simulink model "LineDetectionDSK6416"  (Simulink 6.5)
settings: Solver=FixedStepDiscrete  SolverMode=SingleTasking  StartTime=0.0  StopTime=inf  RelTol=1e-3
libraries: rtdxBlocks x2, viptransforms x2, dspindex x2, c6000tgtpreflib x1, vipconversions x1, vipanalysis x1, vipstatistics x1, viptextngfix x1
settings Model: Creator=jfaing  LastModifiedBy=JacobF  ProdHWDeviceType=TI C6000
settings SolverCC: PositivePriorityOrder=on
settings DataIOCC: SaveOutput=off  SaveTime=off
settings OptimizationCC: OptimizeModelRefInitCode=on
settings HardwareCC: ProdBitPerLong=40  ProdIntDivRoundTo=Zero  ProdEndianess=LittleEndian  ProdHWDeviceType=TI C6000  TargetHWDeviceType=32-bit Generic
settings RTWCC: SystemTargetFile=ti_c6000_ert.tlc  GenCodeOnly=on  TemplateMakefile=ti_c6000_ert.tmf  Description=Embedded Target for TI C6000 DSP (ERT)  ProcessScript=ti_c6000_ert_make_rtw_hook
settings CodeAppCC: IgnoreCustomStorageClasses=off
settings C6000ERTTargetCC: TargetFcnLib=ansi_tfl_tmw.mat  GenFloatMathFcnCalls=ANSI_C  UtilityFuncGeneration=Auto  GenerateFullHeader=on  GenerateSampleERTMain=off  GenerateTestInterfaces=off  IsPILTarget=off  ModelReferenceCompliant=on  IncludeMdlTerminateFcn=on  CombineOutputUpdateFcns=on  SuppressErrorStatus=off  IncludeFileDelimiter=Auto  ERTCustomFileBanners=on  SupportAbsoluteTime=on  LogVarNameModifier=rt_  MatFileLogging=off  MultiInstanceERTCode=off  SupportNonFinite=on  SupportComplex=on  PurelyIntegerCode=off  SupportContinuousTime=off  SupportNonInlinedSFcns=off  EnableShiftOperators=on  ParenthesesLevel=Nominal  GenerateErtSFunction=off  GenerateASAP2=off  ExtMode=off  ExtModeTransport=0  ExtModeStaticAlloc=off  ExtModeStaticAllocSize=1000000  ExtModeTesting=off  ExtModeMexFile=ext_comm  InlinedParameterPlacement=NonHierarchical  TargetOS=BareBoardExample  MultiInstanceErrorCode=Error  RateGroupingCode=on  RootIOFormat=Individual arguments  RTWCAPISignals=off  RTWCAPIParams=off  RTWCAPIStates=off  ERTSrcFileBannerTemplate=ert_code_template.cgt  ERTHdrFileBannerTemplate=ert_code_template.cgt  ERTDataSrcFileTemplate=ert_code_template.cgt  ERTDataHdrFileTemplate=ert_code_template.cgt  ERTCustomFileTemplate=example_file_process.tlc  ModuleNamingRule=Unspecified  SignalDisplayLevel=10  ParamTuneLevel=10  GlobalDataDefinition=Auto  DataDefinitionFile=global.c  GlobalDataReference=Auto  DataReferenceFile=global.h  GRTInterface=off  EnableUserReplacementTypes=off  MemSecPackage=--- None ---  MemSecDataConstants=Default  MemSecDataIO=Default  MemSecDataInternal=Default  MemSecDataParameters=Default  MemSecFuncInitTerm=Default  MemSecFuncExecute=Default  exportCCSObj=on  ccsObjName=CCS_Obj  useDSPBIOS=off  ProfileGenCode=off  InlineDSPBlks=on  FPopt=off  memModel=Far_Aggregate  optLevel=Function(-o2)  CompilerVerbosity=Quiet  InterruptThreshOnC6x=off  SymbolicDebugOnC6x=off  RetainAsmFiles=off  RetainObjFiles=off  CreateMapFile=off  UserStackSize=8192  c6000BuildAction=Create_CCS_Project  OverrunAction=Notify_and_continue  OverrunNotificationMethod=Turn_on_LEDs

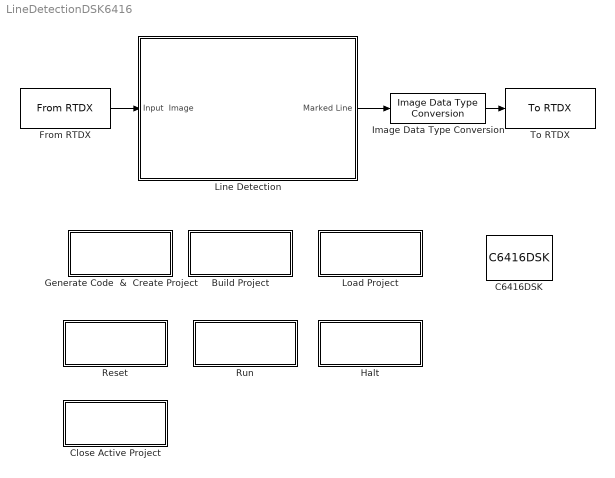
== system LineDetectionDSK6416 ==
  Build Project : Subsystem
      settings: OpenFcn=CCS_Obj.build;
      mask Display: disp('Build\nProject')
  C6416DSK : c6000tgtpreflib/C6416DSK  Tag=C6000 TARGET PREFERENCES BLOCK  SystemSampleTime=-1
  Close Active Project : Subsystem
      settings: OpenFcn=close(CCS_Obj,[],'project')
      mask Display: disp('Close Active Project')
  From RTDX : rtdxBlocks/From RTDX  channelNameStr=inputimage  isBlocking=on  icMaskVar=0  Ts=-1  dims=[99 101]  isFrame=off  dType=uint8  isChannelEnabled=on  isHighSpeedRTDXUsed=on
  Generate Code  &  Create Project : Subsystem
      settings: OpenFcn=make_rtw;
      mask Display: disp('Generate Code\n & \nCreate Project')
  Halt : Subsystem
      settings: OpenFcn=CCS_Obj.halt;
      mask Display: disp('Halt')
  Image Data Type Conversion : vipconversions/Image Data Type Conversion  outDT=uint8  isSigned=on  wordLen=16  numFracBits=0
  Line Detection : Subsystem
  Load Project : Subsystem
      settings: OpenFcn=CCS_Obj.load([pwd,'\',bdroot,'_c6000_rtw\', bdroot, '.out'])
      mask Display: disp('Load\nProject')
  Reset : Subsystem
      settings: OpenFcn=CCS_Obj.reset;
      mask Display: disp('Reset')
  Run : Subsystem
      settings: OpenFcn=CCS_Obj.run;
      mask Display: disp('Run')
  To RTDX : rtdxBlocks/To RTDX  channelNameStr=outputimage  isBlocking=on  isChannelEnabled=on
  wires:
  Image Data Type Conversion/1 -> To RTDX/1
  From RTDX/1 -> Line Detection/1(Input  Image)
  Line Detection/1(Marked Line) -> Image Data Type Conversion/1

== system LineDetectionDSK6416/Build Project ==

== system LineDetectionDSK6416/Close Active Project ==

== system LineDetectionDSK6416/Generate Code  &  Create Project ==

== system LineDetectionDSK6416/Halt ==

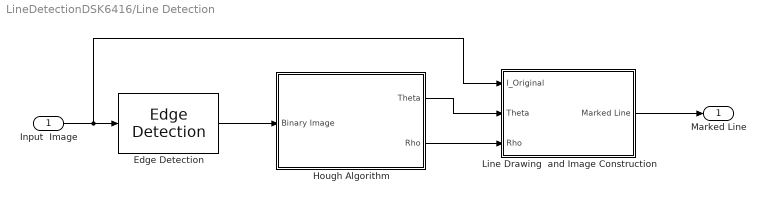
== system LineDetectionDSK6416/Line Detection ==
  Input  Image : Inport
  Edge Detection : vipanalysis/Edge Detection  DialogController=vipDDGCreate  DialogControllerArgs=DataTag1  method=Sobel  outputType=Binary image  userDefinedThreshold=on  thresholdSource=Specify via dialog  threshold=20  thresholdTuning=4  edgeThinning=off  threshold_canny=[0.25 0.60]  autoPercent=70  sigma=1  prodOutputMode=Binary point scaling  prodOutputWordLength=32  prodOutputFracLength=8  roundingMode=Floor  overflowMode=off
  Hough Algorithm : Subsystem
  Line Drawing  and Image Construction : Subsystem
  Marked Line : Outport
  wires:
  Edge Detection/1 -> Hough Algorithm/1(Binary Image)
  Hough Algorithm/2(Rho) -> Line Drawing  and Image Construction/3(Rho)
  Line Drawing  and Image Construction/1(Marked Line) -> Marked Line/1
  Hough Algorithm/1(Theta) -> Line Drawing  and Image Construction/2(Theta)
  Input  Image/1 -> Edge Detection/1, Line Drawing  and Image Construction/1(I_Original)

== system LineDetectionDSK6416/Load Project ==

== system LineDetectionDSK6416/Reset ==

== system LineDetectionDSK6416/Run ==

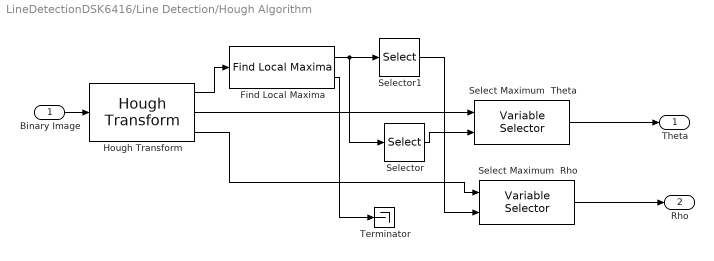
== system LineDetectionDSK6416/Line Detection/Hough Algorithm ==
  Binary Image : Inport
  Find Local Maxima : vipstatistics/Find Local Maxima  num_peaks=1  nhood_size=[5 7]  src_thresh=Specify via dialog  threshold=10  inputIsHough=on  dt_peak=uint32  dt_count=uint32
  Hough Transform : viptransforms/Hough Transform  DialogController=vipDDGCreate  DialogControllerArgs=DataTag2  theta_res=pi/360  rho_res=1  out_theta_rho=on  outdtmode=double  firstCoeffMode=Binary point scaling  firstCoeffWordLength=16  firstCoeffFracLength=14  secondCoeffMode=Binary point scaling  secondCoeffWordLength=32  secondCoeffFracLength=16  outputMode=Binary point scaling  outputWordLength=16  outputFracLength=0  accumMode=Binary point scaling  accumWordLength=32  accumFracLength=20  prodOutputMode=Binary point scaling  prodOutputWordLength=32  prodOutputFracLength=20  memoryMode=Binary point scaling  memoryWordLength=32  memoryFracLength=16  roundingMode=Nearest  overflowMode=on
  Select Maximum  Rho : dspindex/Variable Selector  NumInputs=1  rowsOrCols=Columns  IdxMode=Variable  Elements=[1 3]  ZerOneIdxMode=Zero-based  errmode=Clip Index  FillMode=on  FillValues=0
  Select Maximum  Theta : dspindex/Variable Selector  NumInputs=1  rowsOrCols=Columns  IdxMode=Variable  Elements=[1 3]  ZerOneIdxMode=Zero-based  errmode=Clip Index  FillMode=on  FillValues=0
  Selector : Selector  InputType=Vector  IndexMode=Zero-based  ElementSrc=Internal  Elements=1  RowSrc=Internal  Rows=1  ColumnSrc=Internal  Columns=1  InputPortWidth=2  IndexIsStartValue=off
  Selector1 : Selector  InputType=Vector  IndexMode=Zero-based  ElementSrc=Internal  Elements=0  RowSrc=Internal  Rows=1  ColumnSrc=Internal  Columns=1  InputPortWidth=2  IndexIsStartValue=off
  Terminator : Terminator
  Theta : Outport
  Rho : Outport  Port=2
  wires:
  Find Local Maxima/1 -> Selector1/1, Selector/1
  Find Local Maxima/2 -> Terminator/1
  Selector1/1 -> Select Maximum  Rho/2
  Selector/1 -> Select Maximum  Theta/2
  Hough Transform/3 -> Select Maximum  Rho/1
  Hough Transform/1 -> Find Local Maxima/1
  Hough Transform/2 -> Select Maximum  Theta/1
  Binary Image/1 -> Hough Transform/1
  Select Maximum  Theta/1 -> Theta/1
  Select Maximum  Rho/1 -> Rho/1

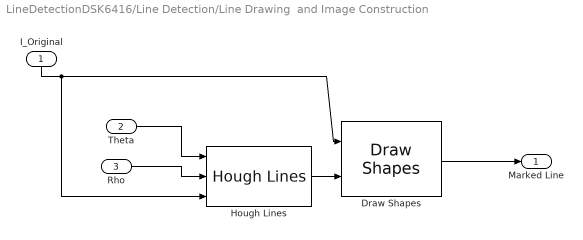
== system LineDetectionDSK6416/Line Detection/Line Drawing  and Image Construction ==
  I_Original : Inport  Orientation=down
  Theta : Inport  Port=2
  Rho : Inport  Port=3
  Draw Shapes : viptextngfix/Draw Shapes  DialogController=vipDDGCreate  DialogControllerArgs=DataTag3  inType=Intensity  shape=Lines  fill=off  display=White  intensity=200  color=[200 255 100]  opacity=0.6  viewport=Entire image  antialiasing=off
  Hough Lines : viptransforms/Hough Lines  DialogController=vipDDGCreate  DialogControllerArgs=DataTag4  sineCompMethod=Trigonometric function  thetaRes=pi/180  firstCoeffMode=Specify word length  firstCoeffWordLength=16  firstCoeffFracLength=15  prodOutputMode=Binary point scaling  prodOutputWordLength=32  prodOutputFracLength=16  roundingMode=Nearest  overflowMode=on
  Marked Line : Outport
  wires:
  Hough Lines/1 -> Draw Shapes/2
  I_Original/1 -> Draw Shapes/1, Hough Lines/3
  Theta/1 -> Hough Lines/1
  Draw Shapes/1 -> Marked Line/1
  Rho/1 -> Hough Lines/2
